simulink model "LKAS_AutoSave_DF_20220316_0937"  (R2018b)
settings: Solver=FixedStepDiscrete  StartTime=0.0  StopTime=10.0  FixedStep=0.01  RelTol=1e-3
InitFcn:
  | tmpVer = ver('MATLAB');
  | tmpVer = str2num(tmpVer.Version);
  | % -------------------------------------------------------------------
  | %  MATLAB file generated by Simulink.saveVars on 21-Nov-2019 10:06:14
  | %  MATLAB version: 7.13.0.564 (R2011b)
  | % -------------------------------------------------------------------
  | 
  | 
  | SInt16 = Simulink.AliasType;
  | SInt16.Description = 'Num';
  | if (tmpVer > 7.11)
  | 	SInt16.DataScope = 'Auto';
  | end
  | SInt16.HeaderFile = 'Rte_Type.h';
  | SInt16.BaseType = 'int16';
  | 
  | SInt32 = Simulink.AliasType;
  | SInt32.Description = 'Num';
  | if (tmpVer > 7.11)
  | 	SInt32.DataScope = 'Auto';
  | end
  | SInt32.HeaderFile = 'Rte_Type.h';
  | SInt32.BaseType = 'int32';
  | 
  | SInt8 = Simulink.AliasType;
  | SInt8.Description = 'Num';
  | if (tmpVer > 7.11)
  | 	SInt8.DataScope = 'Auto';
  | end
  | SInt8.HeaderFile = 'Rte_Type.h';
  | SInt8.BaseType = 'int8';
  | 
  | T_A_m2_1024_1_u32 = Simulink.NumericType;
  | T_A_m2_1024_1_u32.Description = 'm2 (square meters  (m2))';
  | if (tmpVer > 7.11)
  | 	T_A_m2_1024_1_u32.DataScope = 'Auto';
  | end
  | T_A_m2_1024_1_u32.HeaderFile = 'Rte_Type.h';
  | T_A_m2_1024_1_u32.DataTypeMode = 'Fixed-point: slope and bias scaling';
  | T_A_m2_1024_1_u32.SignednessBool = false;
  | T_A_m2_1024_1_u32.WordLength = 32;
  | T_A_m2_1024_1_u32.FixedExponent = -10;
  | T_A_m2_1024_1_u32.SlopeAdjustmentFactor = 1;
  | T_A_m2_1024_1_u32.Bias = 0;
  | T_A_m2_1024_1_u32.DataTypeOverride = 'Inherit';
  | T_A_m2_1024_1_u32.IsAlias = true;
  | 
  | T_A_m2_65536_1_u16 = Simulink.NumericType;
  | T_A_m2_65536_1_u16.Description = 'm2 (square meters  (m2))';
  | if (tmpVer > 7.11)
  | 	T_A_m2_65536_1_u16.DataScope = 'Auto';
  | end
  | T_A_m2_65536_1_u16.HeaderFile = 'Rte_Type.h';
  | T_A_m2_65536_1_u16.DataTypeMode = 'Fixed-point: slope and bias scaling';
  | T_A_m2_65536_1_u16.SignednessBool = false;
  | T_A_m2_65536_1_u16.WordLength = 16;
  | T_A_m2_65536_1_u16.FixedExponent = -16;
  | T_A_m2_65536_1_u16.SlopeAdjustmentFactor = 1;
  | T_A_m2_65536_1_u16.Bias = 0;
  | T_A_m2_65536_1_u16.DataTypeOverride = 'Inherit';
  | ... (+4647 lines)
StopFcn:
  | clear  T_A_m2_1024_1_u32 T_A_m2_65536_1_u16 T_A_m2_Float32 T_A_mm2_10_1_u16 T_A_mm2_4_1_s16 T_A_mm2_Float32 T_Cnt_Num_10_1_u32 T_Cnt_Num_1_1_s16 T_Cnt_Num_1_1_s32 T_Cnt_Num_1_1_s8 T_Cnt_Num_1_1_u16 T_Cnt_Num_1_1_u32 T_Cnt_Num_1_1_u8 T_E_J_1_1_s32 T_E_J_Float32 T_E_kJ_128_1_s32 T_E_kJ_Float32 T_E_kwh_10_1_u16 T_E_kwh_Float32 T_Epl_kwhpkm_100_1_u16 T_Epl_kwhpkm_Float32 T_F_N_1_1_s16 T_F_N_Float32 T_I_A_1000_1_u16 T_I_A_1048576_1_s32 T_I_A_2048_1_s16 T_I_A_32_1_s16 T_I_A_Float32 T_I_mA_1_1_s16 T_I_mA_32768_128_s16 T_I_mA_Float32 T_J_kgpm2_128_1_u16 T_J_kgpm2_Float32 T_K_NA_1000_1_s16 T_K_NA_100_1_s16 T_K_NA_100_1_u16 T_K_NA_1024_1_s16 T_K_NA_1024_1_u16 T_K_NA_128_1_s16 T_K_NA_128_1_u16 T_K_NA_128_1_u8 T_K_NA_16777216_1_u32 T_K_NA_16_1_s16 T_K_NA_16_1_u16 T_K_NA_16_1_u8 T_K_NA_1_16_u16 T_K_NA_1_1_s16 T_K_NA_1_1_u16 T_K_NA_1_1_u8 T_K_NA_32768_1_s16 T_K_NA_32768_1_u16 T_K_NA_32_1_s8 T_K_NA_4096_1_u16 T_K_NA_4194304_1_s32 T_K_NA_4194304_1_u16 T_K_NA_65536_1_s32 T_K_NA_65536_1_u16 T_K_NA_8192_1_s16 T_K_NA_8_1_s16 T_K_NA_Float32 T_M_Nm_16_1_s16 T_M_Nm_1_1_s16 T_M_Nm_32768_1_s16 T_M_Nm_32_1_s16 T_M_Nm_4_1_s16 T_M_Nm_512_1_s16 T_M_Nm_Float32 T_P_W_1_4_s16 T_P_W_1_8_s16 T_P_W_Float32 T_P_kW_128_1_s16 T_P_kW_1_8_s16 T_P_kW_8_1_s32 T_P_kW_Float32 T_Pct_pct_1024_1_s32 T_Pct_pct_1024_1_u32 T_Pct_pct_10_1_s16 T_Pct_pct_10_1_u32 T_Pct_pct_128_100_s8 T_Pct_pct_1_1_s16 T_Pct_pct_1_4_u8 T_Pct_pct_255_100_u16 T_Pct_pct_255_100_u8 T_Pct_pct_256_1_s16 T_Pct_pct_256_1_u16 T_Pct_pct_65535_100_u16 T_Pct_pct_Float32 T_R_ohm_1024_1_s16 T_R_ohm_32_1_s16 T_R_ohm_Float32 T_TK_K_16_1_s16 T_TK_K_Float32 T_T_degC_10_400_1_u16 T_T_degC_16_1_s16 T_T_degC_1_40_1_u8 T_T_degC_2_80_1_u8 T_T_degC_Float32 T_U_V_1000_1_u16 T_U_V_10_1_u8 T_U_V_200_1_u8 T_U_V_32_1_s16 T_U_V_4096_1_s16 T_U_V_512_1_s16 T_U_V_65535_8_u16 T_U_V_8192_1_u16 T_U_V_Float32 T_U_mV_1_1_s16 T_U_mV_256_20_u16 T_U_mV_Float32 T_V_l_256_1_s16 T_V_l_4096_1_s16 T_V_l_64_1_s16 T_V_l_65535_100_u16 T_V_l_Float32 T_V_ml_128_1_s16 T_V_ml_1_1_s16 T_V_ml_32768_1_s16 T_V_ml_Float32 T_V_ul_32_1_u16 T_V_ul_Float32 T_Vpl_clpkm_512_1_u16 T_Vpl_clpkm_Float32 T_a_kphps_16_1_s16 T_a_kphps_Float32 T_a_mps2_128_1_s16 T_a_mps2_Float32 T_c_MJpkg_256_1_s16 T_c_MJpkg_Float32 T_c_kJpgpK_1024_1_s16 T_c_kJpgpK_Float32 T_c_kJpkgpK_128_1_u16 T_c_kJpkgpK_Float32 T_chrg_Ah_1_1_s16 T_chrg_Ah_1_1_u16 T_chrg_Ah_1_1_u8 T_chrg_Ah_256_1_u16 T_chrg_Ah_4194304_1_s32 T_chrg_Ah_512_1_u16 T_chrg_Ah_8_1_u16 T_chrg_Ah_Float32 T_cmp_NA_100_1_s16 T_cmp_NA_128_1_s16 T_cmp_NA_16_1_s16 T_cmp_NA_32768_1_u16 T_cmp_NA_Float32 T_d2n_rpmps2_4_1_s16 T_d2n_rpmps2_Float32 T_dPct_pctps_16_1_s16 T_dPct_pctps_256_1_s16 T_dPct_pctps_Float32 T_dT_degCps_128_1_s16 T_dT_degCps_Float32 T_dV_lph_1_1_s16 T_dV_lph_Float32 T_dV_lpm_128_1_s16 T_dV_lpm_32_1_s16 T_dV_lpm_Float32 T_dV_lps_1024_1_u16 T_dV_lps_4_1_u16 T_dV_lps_Float32 T_dV_mlps_1024_1_s16 T_dV_mlps_Float32 T_d_BitField16 T_dm_gps_128_1_s16 T_dm_gps_128_1_u16 T_dm_gps_256_1_u16 T_dm_gps_Float32 T_dm_mgps_1_1_s16 T_dm_mgps_Float32 T_dn_rpmps_1_1_s16 T_dn_rpmps_2_1_s16 T_dn_rpmps_Float32 T_dp_Paps_1_1_s16 T_dp_Paps_Float32 T_dp_kPaps_1_1_s16 T_dp_kPaps_8_1_s16 T_dp_kPaps_Float32 T_dphi_degps_128_1_s16 T_dphi_degps_8_1_s16 T_dphi_degps_Float32 T_dr_ps_256_1_s16 T_dr_ps_Float32 T_drho_mgplps_1_2_s16 T_drho_mgplps_Float32 T_e_NA_1_1_u8 T_f_Hz_1_1_u16 T_f_Hz_1_1_u32 T_f_Hz_64_1_u16 T_f_Hz_8_1_s16 T_f_Hz_Float32 T_g_BitField32 T_l_km_16_1_s16 T_l_km_1_1_u16 T_l_km_1_1_u32 T_l_km_Float32 T_l_m_1024_1_s16 T_l_m_16_1_s16 T_l_m_1_1_u32 T_l_m_Float32 T_l_mm_16_1_s16 T_l_mm_1_1_u16 T_l_mm_4096_1_s16 T_l_mm_4_1_u8 T_l_mm_64_1_s16 T_l_mm_Float32 T_m_g_1_1_s16 T_m_g_2048_1_s16 T_m_g_32_1_u16 T_m_g_Float32 T_m_kg_1024_1_s16 T_m_kg_1_1_s16 T_m_kg_1_1_u32 T_m_kg_Float32 T_m_mg_128_1_s16 T_m_mg_32_1_s16 T_m_mg_Float32 T_n_rpm_1_1_s16 T_n_rpm_1_25_u8 T_n_rpm_256_50_u16 T_n_rpm_2_25_u8 T_n_rpm_4_1_u16 T_n_rpm_Float32 T_p_MPa_64_1_s16 T_p_MPa_Float32 T_p_Pa_1_1_s16 T_p_Pa_Float32 T_p_kPa_1_10_u16 T_p_kPa_1_1_s16 T_p_kPa_1_1_u8 T_p_kPa_256_1_u16 T_p_kPa_32_1_u16 T_p_kPa_64_1_s16 T_p_kPa_Float32 T_phi_deg_100_1_s16 T_phi_deg_1024_1_s16 T_phi_deg_128_1_s16 T_phi_deg_1_1_u8 T_phi_deg_256_1_s16 T_phi_deg_2_1_s8 T_phi_deg_32_1_s16 T_phi_deg_512_6_s32 T_phi_deg_Float32 T_phi_rad_2048_1_s16 T_phi_rad_Float32 T_r_NA_1024_1_s16 T_r_NA_1024_1_u16 T_r_NA_16384_1_s16 T_r_NA_16_1_s16 T_r_NA_256_1_s8 T_r_NA_256_1_u16 T_r_NA_32768_1_u16 T_r_NA_32_1_u16 T_r_NA_4096_1_s16 T_r_NA_65535_2_u16 T_r_NA_8192_1_u16 T_r_NA_Float32 T_rho_gpl_8192_1_s16 T_rho_gpl_Float32 T_rho_kgpm3_16_1_s16 T_rho_kgpm3_Float32 T_rho_mgpl_1_1_s16 T_rho_mgpl_64_1_s16 T_rho_mgpl_Float32 T_t_hour_1_1_s16 T_t_hour_Float32 T_t_m_1_1_u16 T_t_m_Float32 T_t_ms_1_1_s16 T_t_ms_1_1_u16 T_t_ms_1_1_u32 T_t_ms_4096_1_s16 T_t_ms_64_1_s16 T_t_ms_Float32 T_t_s_1000_1_s16 T_t_s_100_1_s16 T_t_s_10_1_s16 T_t_s_10_1_u16 T_t_s_1_1_s16 T_t_s_1_1_u16 T_t_s_1_1_u32 T_t_s_Float32 T_t_us_10_1_u32 T_t_us_1_1_s16 T_t_us_1_1_u32 T_t_us_1_4_u16 T_t_us_Float32 T_v_kph_1_1_u8 T_v_kph_64_1_s16 T_v_kph_64_1_u16 T_v_kph_Float32 T_v_mps_256_1_s16 T_v_mps_Float32 T_w_radps_32_1_s16 T_w_radps_Float32 T_y_BitField8 T_y_BitFieldDiagProgress T_y_BitFieldDiagStatus T_y_NA_1_1_u8 SInt16 SInt32 SInt8 T_BOOLEAN UInt16 UInt32 UInt8 s16 s32 s8 u16 u32 u8
model workspace (MAT data in the model file):
  MCOS : class17 (value not decoded)
  MCOS : class17 (value not decoded)
  MCOS : class17 (value not decoded)
  MCOS : class17 (value not decoded)
  MCOS : class17 (value not decoded)
  MCOS : class17 (value not decoded)
  MCOS : class17 (value not decoded)
  MCOS : class17 (value not decoded)
  MCOS : class17 (value not decoded)
  MCOS : class17 (value not decoded)
  MCOS : class17 (value not decoded)
  MCOS : class17 (value not decoded)
  MCOS : class17 (value not decoded)
  MCOS : class17 (value not decoded)
  MCOS : class17 (value not decoded)
  MCOS : class17 (value not decoded)
  MCOS : class17 (value not decoded)
  MCOS : class17 (value not decoded)
  MCOS : class17 (value not decoded)
  MCOS : class17 (value not decoded)
  MCOS : class17 (value not decoded)
  MCOS : class17 (value not decoded)
  MCOS : class17 (value not decoded)
  MCOS : class17 (value not decoded)
  MCOS : class17 (value not decoded)
  MCOS : class17 (value not decoded)
  MCOS : class17 (value not decoded)
  MCOS : class17 (value not decoded)
  MCOS : class17 (value not decoded)
  MCOS : class17 (value not decoded)
  MCOS : class17 (value not decoded)
  MCOS : class17 (value not decoded)
  MCOS : class17 (value not decoded)
  MCOS : class17 (value not decoded)
  MCOS : class17 (value not decoded)
  MCOS : class17 (value not decoded)
  MCOS : class17 (value not decoded)
  MCOS : class17 (value not decoded)
  MCOS : class17 (value not decoded)
  MCOS : class17 (value not decoded)
  MCOS : class17 (value not decoded)
  MCOS : class17 (value not decoded)
  MCOS : class17 (value not decoded)
  MCOS : class17 (value not decoded)
  MCOS : class17 (value not decoded)
  MCOS : class17 (value not decoded)
  MCOS : class17 (value not decoded)
  MCOS : class17 (value not decoded)
  MCOS : class17 (value not decoded)
  MCOS : class17 (value not decoded)
  MCOS : class17 (value not decoded)
  MCOS : class17 (value not decoded)
  MCOS : class17 (value not decoded)
  MCOS : class17 (value not decoded)
  MCOS : class17 (value not decoded)
  MCOS : class17 (value not decoded)
  MCOS : class17 (value not decoded)
  MCOS : class17 (value not decoded)
  MCOS : class17 (value not decoded)
  MCOS : class17 (value not decoded)
  MCOS : class17 (value not decoded)
  MCOS : class17 (value not decoded)
  MCOS : class17 (value not decoded)
  MCOS : class17 (value not decoded)
  MCOS : class17 (value not decoded)
  MCOS : class17 (value not decoded)
  MCOS : class17 (value not decoded)
  MCOS : class17 (value not decoded)
  MCOS : class17 (value not decoded)
  MCOS : class17 (value not decoded)
  MCOS : class17 (value not decoded)
  MCOS : class17 (value not decoded)
  MCOS : class17 (value not decoded)
  MCOS : class17 (value not decoded)
  MCOS : class17 (value not decoded)
  MCOS : class17 (value not decoded)
  MCOS : class17 (value not decoded)
  MCOS : class17 (value not decoded)
  MCOS : class17 (value not decoded)
  MCOS : class17 (value not decoded)
  MCOS : class17 (value not decoded)
  MCOS : class17 (value not decoded)
  MCOS : class17 (value not decoded)
  MCOS : class17 (value not decoded)
  MCOS : class17 (value not decoded)
  MCOS : class17 (value not decoded)
  MCOS : class17 (value not decoded)
  MCOS : class17 (value not decoded)
  MCOS : class17 (value not decoded)
  MCOS : class17 (value not decoded)
  MCOS : class17 (value not decoded)
  MCOS : class17 (value not decoded)
  MCOS : class17 (value not decoded)
  MCOS : class17 (value not decoded)
  MCOS : class17 (value not decoded)
  MCOS : class17 (value not decoded)
  MCOS : class17 (value not decoded)
  MCOS : class17 (value not decoded)
  MCOS : class17 (value not decoded)
  MCOS : class17 (value not decoded)
  MCOS : class17 (value not decoded)
  MCOS : class17 (value not decoded)
  MCOS : class17 (value not decoded)
  MCOS : class17 (value not decoded)
  MCOS : class17 (value not decoded)
undefined symbols (not defined in the file): LKA_CarWidth, LKA_SampleTime, LKA_StrRatio_C, LKA_Veh2CamL_C, LKA_Veh2CamW_C, LKA_WhlBaseL_C, LL_CompHdAg_C, LL_CompSWA_C, LL_CrvtPrvwT_C, LL_DesDvt_C, LL_DvtComp_C, LL_DvtPrvwT_C, LL_DvtSpdDet_vDvtSpdMin_C, LL_HandsOff_ExitTime, LL_HandsOff_TextTime, LL_HandsOff_WarnTime, LL_HdAgExT_C, LL_HdAgPrvwT_C, LL_LAccMax_C, LL_LAccRMax_C, LL_LDW_EarliestWarnLine_C, LL_LDW_LatestWarnLine_C, LL_LDWS_SUPPRESS_HEADING, LL_LFClb_TFC_FfCtlRatio_C, LL_LFClb_TFC_KdBalance_C, LL_LFClb_TFC_KdMaxSWA_C, LL_LFClb_TFC_KdV1_C, LL_LFClb_TFC_KdV2_C, LL_LFClb_TFC_KdVehSpdLwr_C, LL_LFClb_TFC_KdVehSpdUpr_C, LL_LFClb_TFC_Ki_C, LL_LFClb_TFC_KiMaxSWA_C, LL_LFClb_TFC_Kp_C, LL_LFClb_TFC_KpKlat_C, LL_LFClb_TFC_KpV1_C, LL_LFClb_TFC_KpV2_C, LL_LFClb_TFC_KpVehSpdLwr_C, LL_LFClb_TFC_KpVehSpdUpr_C, LL_LFClb_TFC_PrvwT_C, LL_LKA_EarliestWarnLine_C, LL_LKA_LatestWarnLine_C, LL_LKAExPrcs_ExitC0Dvt, LL_LKAExPrcs_ExitC0Swt, LL_LKAExPrcs_tiExitDelayTime3, LL_LKAExPrcs_tiExitTime1, LL_LKAExPrcs_tiExitTime2, LL_LKAExPrcs_tiExitTime3, LL_LKAS_OUT_OF_CONTROL_LAT_VEL, LL_LKAS_OUT_OF_CONTROL_TTLC, LL_LKASWASyn_M0, LL_LKASWASyn_M1, LL_LKASWASyn_M2, LL_LKASWASyn_M3D, LL_LKASWASyn_M3K_DT, LL_LKASWASyn_M3K_MSD, LL_LKASWASyn_SWAaddMax, LL_LKASWASyn_T2, LL_LKASWASyn_tiTrqSwaRtTime, LL_LKASWASyn_tiTrqSwaTime, LL_LKASWASyn_TrqMax ... (+46)
libraries: simulink x139, canmsglib x8, dspstat3 x3, simulink_extras x1
(part 7 of 20)

== system LKAS_AutoSave_DF_20220316_0937/LKAS/LL/LL Inputs Mapping/bsVehMovInfo ==
  bsVehMovInfoIn : Inport
  Bus Creator : BusCreator  Inputs=10
  Bus Selector2 : BusSelector  OutputSignals=ESC_LatAcc,ESC_LatAcc_Valid,ESC_YawRate,ESC_YawRate_Valid,ESC_UnYawRate,ESC_VehSpd,ESC_LonAcc,ESC_LonAcc_Valid,ESC_Brake_Press,ESC_VehSpd_Valid
  bsVehMovInfoOut : Outport
  wires:
  Bus Creator/1 -> bsVehMovInfoOut/1
  Bus Selector2/10 -> Bus Creator/10  "<ESC_VehSpd_Valid>"
  Bus Selector2/9 -> Bus Creator/9  "<ESC_Brake_Press>"
  Bus Selector2/8 -> Bus Creator/8  "<ESC_LonAcc_Valid>"
  Bus Selector2/7 -> Bus Creator/7  "<ESC_LonAcc>"
  Bus Selector2/6 -> Bus Creator/6  "<ESC_VehSpd>"
  Bus Selector2/5 -> Bus Creator/5  "<ESC_UnYawRate>"
  Bus Selector2/4 -> Bus Creator/4  "<ESC_YawRate_Valid>"
  Bus Selector2/3 -> Bus Creator/3  "<ESC_YawRate>"
  Bus Selector2/2 -> Bus Creator/2  "<ESC_LatAcc_Valid>"
  Bus Selector2/1 -> Bus Creator/1  "<ESC_LatAcc>"
  bsVehMovInfoIn/1 -> Bus Selector2/1

== system LKAS_AutoSave_DF_20220316_0937/LKAS/LL/LLOn/LDW ==
  LDW_bsLKAInfoSyn : Inport
  LDW_bsLDWClb : Inport  Port=2
  Enable : EnablePort  StatesWhenEnabling=reset  ShowOutputPort=on
      settings: AttributesFormatString=states = %<StatesWhenEnabling>
  Bus Selector : BusSelector  OutputSignals=bsHdAgInfo.phiHdAg_Lft,bsHdAgInfo.phiHdAg_Rgt
  Bus Selector1 : BusSelector  OutputSignals=bsLDWClb.LL_LDWS_SUPPRESS_HEADING,bsConstantClb.LKA_SampleTime
  Cast : DataTypeConversion  OutDataTypeStr=uint8
  Heading Angle Detection (HdAgDet) : Subsystem  Description=|
      | Block Name: Heading Angle Detection
      | Ab.: HdAgDet
      | No.: 1.3.1.0
      | Rev: 0.0.1
      | Update Date: 19-3-26
  Logical Operator : Logic  Operator=NOT  AllPortsSameDT=off  OutDataTypeStr=boolean
  Product : Product  OutDataTypeStr=uint8
  LDW_Flag : Outport  OutputWhenDisabled=reset  InitialOutput=0
      settings: AttributesFormatString=%<OutputWhenDisabled> = %<InitialOutput>
  wires:
  Logical Operator/1 -> Cast/1
  Cast/1 -> Product/2
  Bus Selector1/2 -> Heading Angle Detection (HdAgDet)/5(SampleTime)  "<LKA_SampleTime>"
  Product/1 -> LDW_Flag/1
  Heading Angle Detection (HdAgDet)/1(HdAgDet_stHdAgDetFlg) -> Logical Operator/1
  LDW_bsLKAInfoSyn/1 -> Bus Selector/1
  Enable/1 -> Heading Angle Detection (HdAgDet)/1(HdAgDet_stLDWActvFlg), Product/1
  Bus Selector/1 -> Heading Angle Detection (HdAgDet)/2(HdAgDet_phiHdAgLft)  "<phiHdAg_Lft>"
  Bus Selector/2 -> Heading Angle Detection (HdAgDet)/3(HdAgDet_phiHdAgRgt)  "<phiHdAg_Rgt>"
  LDW_bsLDWClb/1 -> Bus Selector1/1
  Bus Selector1/1 -> Heading Angle Detection (HdAgDet)/4(HdAgDet_phiHdAgThres_C)  "<LL_LDWS_SUPPRESS_HEADING>"

== system LKAS_AutoSave_DF_20220316_0937/LKAS/LL/LLOn/LKA ==
  LKA_bsInInfoSyn : Inport
  LKA_bsLKAInPInfo : Inport  Port=2
  LKA_bsLKAClb : Inport  Port=3
  Enable : EnablePort  StatesWhenEnabling=reset  ShowOutputPort=on
      settings: AttributesFormatString=states = %<StatesWhenEnabling>
  Bus Selector : BusSelector  OutputSignals=bsConstantClb.LKA_SampleTime
  Cast To Single : DataTypeConversion  OutDataTypeStr=uint8
  Driver Torque Addition (DTA) : Subsystem
  LKA Exit Processing (LKAExPrcs) : Subsystem  Description=|
      | Block Name: LKA Exit Processing 
      | Ab.: LKAExPrcs
      | No.: 1.2.2.0
      | Rev: 0.0.1
      | Update Date: 19-5-13
  "LKA Motion Planning (LKAMP) " : Subsystem  Description=|
      | Block Name: LKA Motion Planning
      | Ab.: LKAMP
      | No.: 1.2.3.0
      | Rev: 0.0.1
      | Update Date: 19-5-13
  LKA SWA Limit (LKASWALim) : Subsystem  Description=|
      | Block Name: LKA SWA Synthesis
      | Ab.: LKASWASyn
      | No.: 1.2.6.0
      | Rev: 0.0.1
      | Update Date: 19-5-13
  LKA_Mon : Subsystem
  Lane Following (LF) : Subsystem  Description=|
      | Block Name: Lane Following
      | Ab.: LF
      | No.: 02
      | Rev: 00.00.01
      | Update Date: 19-3-28
  Plan To LaneFollowing (PTLF) : Subsystem
  LKA_ExitFlg : Outport  OutputWhenDisabled=reset  InitialOutput=0
      settings: AttributesFormatString=%<OutputWhenDisabled> = %<InitialOutput>
  LKA_phiSWACmd : Outport  Port=2  OutputWhenDisabled=reset  InitialOutput=0
      settings: AttributesFormatString=%<OutputWhenDisabled> = %<InitialOutput>
  LKA_M : Outport  Port=3  OutputWhenDisabled=reset  InitialOutput=0
      settings: AttributesFormatString=%<OutputWhenDisabled> = %<InitialOutput>
  LKAMon : Outport  Port=4  OutputWhenDisabled=reset  InitialOutput=0
      settings: AttributesFormatString=%<OutputWhenDisabled> = %<InitialOutput>
  tag scope: ActFlg=global, Ff=global, LKA_ExitFlg_Mon=global, LKA_SampleTime=global, PT1=global
  wires:
  Cast To Single/1 -> [ActFlg]  "ActFlg"
  Plan To LaneFollowing (PTLF)/1(SWACmd) -> LKA SWA Limit (LKASWALim)/1(LKASWALim_phiTFCSWACmd)  "PTLFSWACmd"
  Enable/1 -> Cast To Single/1
  LKA SWA Limit (LKASWALim)/1(LKASWALim_phiSWACmd) -> LKA_phiSWACmd/1  "phiSWACmd"
  LKA Exit Processing (LKAExPrcs)/1(LKAExPrcs_stExFlg) -> LKA_ExitFlg/1, [LKA_ExitFlg_Mon]
  [Ff] -> Plan To LaneFollowing (PTLF)/5(Ff)
  [P] -> Plan To LaneFollowing (PTLF)/6(P)
  [I] -> Plan To LaneFollowing (PTLF)/7(I)
  [D] -> Plan To LaneFollowing (PTLF)/8(D)
  Driver Torque Addition (DTA)/1(DTA_phiDTASWACmd) -> [DT]  "DT"
  [DT] -> Plan To LaneFollowing (PTLF)/4(DrvTrq)
  [Plan] -> Plan To LaneFollowing (PTLF)/2(Plan)
  [PT1] -> Plan To LaneFollowing (PTLF)/3(T1)
  [PT1] -> LKA Exit Processing (LKAExPrcs)/3(LKAExPrcs_PlanT1)
  [ActFlg] -> "LKA Motion Planning (LKAMP) "/3(LKAMP_stLKAActvFlg)
  LKA_bsLKAInPInfo/1 -> [LKAInPInfo]
  [LKAInPInfo] -> "LKA Motion Planning (LKAMP) "/4(LKAMP_bsLKAInPInfo)
  [LKAInPInfo] -> LKA Exit Processing (LKAExPrcs)/1(LKAExPrcs_bsLKAInPInfo)
  [LKAInPInfo] -> Plan To LaneFollowing (PTLF)/1(InP)
  LKA_bsLKAClb/1 -> Bus Selector/1, [LKA_bsLLClb]
  [LKAInPInfo] -> LKA SWA Limit (LKASWALim)/3(LKASWALim_bsLKAInPInfo)
  [LKA_bsLLClb] -> LKA Exit Processing (LKAExPrcs)/2(LKAExPrcs_bsLKAClb)
  [LKA_bsLLClb] -> Driver Torque Addition (DTA)/2(DTA_bsLFClb)
  [LKA_bsLLClb] -> Lane Following (LF)/3(LF_bsLFClb)
  [LKA_bsLLClb] -> LKA SWA Limit (LKASWALim)/4(LKASWALim_bsLKAClb)
  LKA_bsInInfoSyn/1 -> [LKA_bsInInfoSyn]
  [LKA_bsInInfoSyn] -> "LKA Motion Planning (LKAMP) "/1(LKAMP_bsInInfoSyn)
  [LKA_bsInInfoSyn] -> Driver Torque Addition (DTA)/1(DTA_bsInInfoSyn)
  [LKA_bsInInfoSyn] -> Lane Following (LF)/1(LF_bsInInfoSyn)
  [Ff] -> LKA SWA Limit (LKASWALim)/2(LKASWALim_Ff)
  [LKAInPInfo] -> Lane Following (LF)/2(LF_bsLKAInPInfo)
  Driver Torque Addition (DTA)/2(DTA_M) -> LKA_M/1
  Lane Following (LF)/3(LF_phiIntegSWACmd) -> [I]
  Lane Following (LF)/1(LF_phiFfLFSWACmd) -> [Ff]
  Lane Following (LF)/2(LF_phiPropSWACmd) -> [P]
  Lane Following (LF)/4(LF_phiDiffSWACmd) -> [D]
  "LKA Motion Planning (LKAMP) "/1(LKAMP_phiSWACmd) -> [Plan]  "PlanSWACmd"
  "LKA Motion Planning (LKAMP) "/2(LKAMP_tiT1) -> [PT1]  "PlanT1"
  LKA_Mon/1(LKAMon) -> LKAMon/1
  [LKA_bsLLClb] -> "LKA Motion Planning (LKAMP) "/5(LKAMP_bsLLClb)
  Bus Selector/1 -> [LKA_SampleTime]  "<LKA_SampleTime>"
  [Ff] -> "LKA Motion Planning (LKAMP) "/2(LKAMP_Ff)

== system LKAS_AutoSave_DF_20220316_0937/LKAS/LL/LLOn/LKA Input Processing (LKAInP) ==
  LKAInP_bsInInfoSyn : Inport
  LKAInP_bsLLClb : Inport  Port=2
  LKAInP_ActFlg : Inport  Port=3
  Bus Creator2 : BusCreator  Inputs=10
  Curvature Calculation (Crvt) : Subsystem
  Delay : Delay  DelayLength=1
  Deviation Calculation (Dvt) : Subsystem
  Heading Angle Calculation (HdAg) : Subsystem
  Lane Width Calculation (LW) : Subsystem
  Previewed Curvature Calculation (PrCrvt) : Subsystem
  Previewed Deviation Calculation (PrDvt) : Subsystem
  Previewed Heading Angle Calculation (PrHdAg) : Subsystem
  Steering Wheel Position Calculation (SWAPosCal) : Subsystem
  TTLC Calculation (TTLCCalc) : Subsystem  Description=|
      | Block Name: TTLC Calculation
      | Ab.: TTLCCalc
      | No.: 1.1.1.1
      | Rev: 0.0.1
      | Update Date: 19-3-26
  Under The Limit (UndrLim) : Subsystem
  LKAInP_bsLKAInPInfo : Outport
  wires:
  LKAInP_bsInInfoSyn/1 -> Previewed Heading Angle Calculation (PrHdAg)/1(PrHdAg_bsInInfoSyn), TTLC Calculation (TTLCCalc)/3(TTLCCalc_bsInfo), Previewed Deviation Calculation (PrDvt)/2(PrvwDvt_bsInInfoSyn), Previewed Curvature Calculation (PrCrvt)/1(PrvwCrvt_bsInInfoSyn), Deviation Calculation (Dvt)/1(Dvt_bsInInfoSyn), Heading Angle Calculation (HdAg)/1(HdAg_bsInInfoSyn), Curvature Calculation (Crvt)/1(PrvwCrvt_bsInInfoSyn), Under The Limit (UndrLim)/1(UndrLim_bsInInfoSyn), Lane Width Calculation (LW)/1(LW_bsInInfoSyn), Steering Wheel Position Calculation (SWAPosCal)/1(SWAPosCal_bsInInfoSyn)
  [bsHdAgInfo] -> Bus Creator2/5  "bsHdAgInfo"
  LKAInP_bsLLClb/1 -> Previewed Deviation Calculation (PrDvt)/1(PrdcDvt_bsLLClb), Previewed Heading Angle Calculation (PrHdAg)/2(PrHdAg_bsLLClb), Deviation Calculation (Dvt)/2(Dvt_bsLLClb), Under The Limit (UndrLim)/2(UndrLim_bsLLClb), Steering Wheel Position Calculation (SWAPosCal)/2(SWAPosCal_bsLLClb), Previewed Curvature Calculation (PrCrvt)/2(PrvwCrvt_tiCrvtPrvwT_C), TTLC Calculation (TTLCCalc)/2(TTLCCalc_bsLLClb)
  [bsPrHdAgInfo] -> Bus Creator2/8  "bsPrHdAgInfo"
  [bsTTLCInfo] -> Bus Creator2/10  "bsTTLCInfo"
  [LaneWidth] -> Bus Creator2/1  "LaneWidth"
  [phiSWAPos] -> Bus Creator2/2  "phiSWAPos"
  [bsUndrLimInfo] -> Bus Creator2/3  "bsUndrLimInfo"
  [bsDvtInfo] -> Bus Creator2/6  "bsDvtInfo"
  [bsCrvtInfo] -> Bus Creator2/4  "bsCrvtInfo"
  [bsPrDvtInfo] -> Bus Creator2/9  "bsPrDvtInfo"
  [bsPrCrvtInfo] -> Bus Creator2/7  "bsPrCrvtInfo"
  Bus Creator2/1 -> LKAInP_bsLKAInPInfo/1
  LKAInP_ActFlg/1 -> Delay/1
  Delay/1 -> Previewed Curvature Calculation (PrCrvt)/3(PrvwCrvt_stLKAActvFlg)
  Lane Width Calculation (LW)/1(LW_LaneWidth) -> [LaneWidth]  "LaneWidth"
  Steering Wheel Position Calculation (SWAPosCal)/1(SWAPosCal) -> [phiSWAPos]  "phiSWAPos"
  Under The Limit (UndrLim)/1(UndrLim_bsUndrLimInfo) -> [bsUndrLimInfo]  "bsUndrLimInfo"
  Curvature Calculation (Crvt)/1(Crvt_bsCrvtInfo) -> [bsCrvtInfo]  "bsCrvtInfo"
  Heading Angle Calculation (HdAg)/1(HdAg_bsHdAgInfo) -> [bsHdAgInfo]  "bsHdAgInfo"
  [bsHdAgInfo] -> TTLC Calculation (TTLCCalc)/5(TTLCCalc_bsHdAgInfo)  "bsHdAgInfo"
  Deviation Calculation (Dvt)/1(Dvt_bsDvtInfo) -> [bsDvtInfo]  "bsDvtInfo"
  [bsDvtInfo] -> TTLC Calculation (TTLCCalc)/1(TTLCCalc_bsDvtInfo)  "bsDvtInfo"
  Previewed Curvature Calculation (PrCrvt)/1(PrvwCrvt_bsPrvwCrvtInfo) -> [bsPrCrvtInfo]  "bsPrCrvtInfo"
  [bsPrCrvtInfo] -> TTLC Calculation (TTLCCalc)/4(TTLCCalc_bsPrCrvtInfo)  "bsPrCrvtInfo"
  Previewed Heading Angle Calculation (PrHdAg)/1(PrHdAg_bsPrHdAgInfo) -> [bsPrHdAgInfo]  "bsPrHdAgInfo"
  Previewed Deviation Calculation (PrDvt)/1(PrvwDvt_bsPrvwDvtInfo) -> [bsPrDvtInfo]  "bsPrDvtInfo"
  TTLC Calculation (TTLCCalc)/1(TTLCCalc_bsTTLCInfo) -> [bsTTLCInfo]  "bsTTLCInfo"
  [bsTTLCInfo] -> Previewed Heading Angle Calculation (PrHdAg)/3(PrHdAg_bsTTLCInfo)  "bsTTLCInfo"

== system LKAS_AutoSave_DF_20220316_0937/LKAS/LL/LLOn/LL State Determination (LLStateDet) ==
  LLStateDet_bsInInfoSyn : Inport
  LLStateDet_bsLKAInPInfo : Inport  Port=2
  LLStateDet_bsLLClb : Inport  Port=3
  LLStateDet_stExitFlg : Inport  Port=4
  LLStateDet_SignalFault : Inport  Port=5
  Bus Creator : BusCreator  Inputs=3
  Delay : Delay  DelayLength=1
  Delay1 : Delay  DelayLength=1
  LDW_State_Machine : Stateflow chart  Description=|  TreatAsAtomicUnit=on
      | Block Name: LDW State Machine
      | Ab.: LDWSM
      | No.: 1.1.2.0
      | Rev: 0.0.1
      | Update Date: 19-3-26
      settings: RTWSystemCode=Nonreusable function
  LKA_State_Machine : Stateflow chart  Description=|  TreatAsAtomicUnit=on
      | Block Name: LKA State Machine
      | Ab.: LKASM
      | No.: 1.1.3.0
      | Rev: 0.0.1
      | Update Date: 19-3-26
      settings: RTWSystemCode=Nonreusable function
  LL State Machine Conditions (LLSMCon) : Subsystem
  LLStateDet_bsLLState : Outport
  LLStateDet_stLDWActvFlg : Outport  Port=2
  LLStateDet_stLKAActvFlg : Outport  Port=3
  Disable_Reason : Outport  Port=4
  tag scope: LDW_State_Mon=global, LKA_State_Mon=global
  wires:
  LL State Machine Conditions (LLSMCon)/2(LLSMCon_stLDWEnaCSyn) -> LDW_State_Machine/2(LDWSM_stEnaCSyn)
  LL State Machine Conditions (LLSMCon)/3(LLSMCon_stLDWDisblCSyn) -> LDW_State_Machine/3(LDWSM_stDisblCSyn)
  LL State Machine Conditions (LLSMCon)/4(LLSMCon_stLDWActvCSyn) -> LDW_State_Machine/4(LDWSM_stActvCSyn)
  LL State Machine Conditions (LLSMCon)/5(LLSMCon_stLDWDeactvCSyn) -> LDW_State_Machine/5(LDWSM_stDeactvCSyn)
  LL State Machine Conditions (LLSMCon)/1(LLSMCon_stDACMode) -> Bus Creator/2, LKA_State_Machine/1(LKASM_stLMCMode), LDW_State_Machine/1(LDWSM_stLMCMode)  "DACMode"
  LDW_State_Machine/1(LDWSM_stLDWActvFlg) -> LLStateDet_stLDWActvFlg/1
  LKA_State_Machine/1(LKASM_stLKAActvFlg) -> LLStateDet_stLKAActvFlg/1
  Delay1/1 -> LL State Machine Conditions (LLSMCon)/4(LLSMCon_bsLLState)
  Bus Creator/1 -> LLStateDet_bsLLState/1, Delay1/1  "LLState"
  LKA_State_Machine/2(LKASM_stLKAState) -> [LKA_State_Mon], Bus Creator/3  "LKA_State"
  LDW_State_Machine/2(LDWSM_stLDWState) -> [LDW_State_Mon], Bus Creator/1  "LDW_State"
  LL State Machine Conditions (LLSMCon)/6(LLSMCon_stLDWFaultCSyn) -> LDW_State_Machine/6(LDWSM_stFaultCSyn)
  LL State Machine Conditions (LLSMCon)/7(LLSMCon_stLKAEnaCSyn) -> LKA_State_Machine/2(LKASM_stEnaCSyn)
  LL State Machine Conditions (LLSMCon)/8(LLSMCon_stLKADisblCSyn) -> LKA_State_Machine/3(LKASM_stDisblCSyn)
  LL State Machine Conditions (LLSMCon)/9(LLSMCon_stLKAActvCSyn) -> LKA_State_Machine/4(LKASM_stActvCSyn)
  LL State Machine Conditions (LLSMCon)/10(LLSMCon_stLKADeactvCSyn) -> LKA_State_Machine/5(LKASM_stDeactvCSyn)
  LL State Machine Conditions (LLSMCon)/11(LLSMCon_stLKAFaultCSyn) -> LKA_State_Machine/6(LKASM_stFaultCSyn)
  LLStateDet_bsInInfoSyn/1 -> LL State Machine Conditions (LLSMCon)/1(LLSMCon_bsInInfoSyn)
  LLStateDet_bsLKAInPInfo/1 -> LL State Machine Conditions (LLSMCon)/2(LLSMCon_bsLKAInPInfo)
  LLStateDet_stExitFlg/1 -> Delay/1
  LLStateDet_bsLLClb/1 -> LL State Machine Conditions (LLSMCon)/3(LLSMCon_bsLLClb)
  Delay/1 -> LL State Machine Conditions (LLSMCon)/5(LLSMCon_stExitFlg)
  LLStateDet_SignalFault/1 -> LL State Machine Conditions (LLSMCon)/6(LLSMCon_bsSignalFault)
  LL State Machine Conditions (LLSMCon)/12(Disable_Reason) -> Disable_Reason/1

== system LKAS_AutoSave_DF_20220316_0937/LKAS/LL/LLOn/LL_Mon ==
  Disable_Reason : Inport
  LKAMon : Inport  Port=2
  Bus : BusCreator  Inputs=4
  BusInP : BusCreator  Inputs=2
  BusState : BusCreator  Inputs=2
  LLMon : Outport
  wires:
  [InPMon] -> Bus/1
  [StateMon] -> Bus/2
  LKAMon/1 -> Bus/3
  Bus/1 -> LLMon/1  "LLMon"
  [LFTTTLC_Mon] -> BusInP/1  "LFTTTLC_Mon"
  [RGTTTLC_Mon] -> BusInP/2  "RGTTTLC_Mon"
  [LDW_State_Mon] -> BusState/1  "LDW_State_Mon"
  [LKA_State_Mon] -> BusState/2  "LKA_State_Mon"
  BusInP/1 -> [InPMon]  "InPMon"
  BusState/1 -> [StateMon]  "StateMon"
  Disable_Reason/1 -> Bus/4  "Disable_Reason"

== system LKAS_AutoSave_DF_20220316_0937/LKAS/LL/LLOut/Angle2Trq ==
  LKA_Torque_Req : Inport
  Target_Angle : Inport  Port=2
  Stearing_Angle : Inport  Port=3
  Constant : Constant  Value=5  OutDataTypeStr=single
  Constant1 : Constant  Value=-5  OutDataTypeStr=single
  Constant3 : Constant  Value=5  OutDataTypeStr=single
  Constant4 : Constant  Value=-5  OutDataTypeStr=single
  Rate Limiter Dynamic : Subsystem
  Saturation Dynamic : Subsystem
  Subsystem : Subsystem
  torque : Outport  OutputWhenDisabled=reset  InitialOutput=0
  wires:
  Saturation Dynamic/1(y) -> torque/1  "Saturation_trq"
  Constant4/1 -> Saturation Dynamic/3(lo)
  Constant3/1 -> Saturation Dynamic/1(up)
  Rate Limiter Dynamic/1(Y) -> Saturation Dynamic/2(u)  "RL_trq"
  Constant1/1 -> Rate Limiter Dynamic/3(lo)
  Constant/1 -> Rate Limiter Dynamic/1(up)
  Target_Angle/1 -> Subsystem/1(Target_Angle)  "Target_Angle"
  Stearing_Angle/1 -> Subsystem/2(Stearing_Angle)  "Stearing_Angle"
  Subsystem/1(in_trq) -> Rate Limiter Dynamic/2(u)  "in_trq"
  LKA_Torque_Req/1 -> Subsystem/Enable  "LKA_Torque_Req"

== system LKAS_AutoSave_DF_20220316_0937/LKAS/LLClb/LLSMConClb/ICv to v10 ==
  In1 : Inport
  Add : Sum  Inputs=+-
  Constant : Constant  Value=2.5  OutDataTypeStr=single
  Gain : Gain  Gain=1/1.02
  Out1 : Outport
  wires:
  In1/1 -> Add/1
  Add/1 -> Gain/1
  Constant/1 -> Add/2
  Gain/1 -> Out1/1

== system LKAS_AutoSave_DF_20220316_0937/LKAS/LLClb/LLSMConClb/ICv to v11 ==
  In1 : Inport
  Add : Sum  Inputs=+-
  Constant : Constant  Value=2.5  OutDataTypeStr=single
  Gain : Gain  Gain=1/1.02
  Out1 : Outport
  wires:
  Gain/1 -> Out1/1
  Constant/1 -> Add/2
  Add/1 -> Gain/1
  In1/1 -> Add/1

== system LKAS_AutoSave_DF_20220316_0937/LKAS/LLClb/LLSMConClb/ICv to v6 ==
  In1 : Inport
  Add : Sum  Inputs=+-
  Constant : Constant  Value=2.5  OutDataTypeStr=single
  Gain : Gain  Gain=1/1.02
  Out1 : Outport
  wires:
  In1/1 -> Add/1
  Add/1 -> Gain/1
  Constant/1 -> Add/2
  Gain/1 -> Out1/1

== system LKAS_AutoSave_DF_20220316_0937/LKAS/LLClb/LLSMConClb/ICv to v7 ==
  In1 : Inport
  Add : Sum  Inputs=+-
  Constant : Constant  Value=2.5  OutDataTypeStr=single
  Gain : Gain  Gain=1/1.02
  Out1 : Outport
  wires:
  Gain/1 -> Out1/1
  Constant/1 -> Add/2
  Add/1 -> Gain/1
  In1/1 -> Add/1

== system LKAS_AutoSave_DF_20220316_0937/LKAS/LLClb/LLSMConClb/ICv to v8 ==
  In1 : Inport
  Add : Sum  Inputs=+-
  Constant : Constant  Value=2.5  OutDataTypeStr=single
  Gain : Gain  Gain=1/1.02
  Out1 : Outport
  wires:
  In1/1 -> Add/1
  Add/1 -> Gain/1
  Constant/1 -> Add/2
  Gain/1 -> Out1/1

== system LKAS_AutoSave_DF_20220316_0937/LKAS/LLClb/LLSMConClb/ICv to v9 ==
  In1 : Inport
  Add : Sum  Inputs=+-
  Constant : Constant  Value=2.5  OutDataTypeStr=single
  Gain : Gain  Gain=1/1.02
  Out1 : Outport
  wires:
  Gain/1 -> Out1/1
  Constant/1 -> Add/2
  Add/1 -> Gain/1
  In1/1 -> Add/1

== system LKAS_AutoSave_DF_20220316_0937/LKAS/LL/Human Machine Interface (HMI)/Subsystem/Sum Condition1 ==
  SampleTime : Inport
  Sum : Inport  Port=2
  state = reset : EnablePort  StatesWhenEnabling=reset
  Add1 : Sum  OutDataTypeStr=single
  Memory : Memory  InheritSampleTime=on
  Relational Operator : RelationalOperator  OutDataTypeStr=boolean  RndMeth=Nearest
  Saturation : Saturate  UpperLimit=60  LowerLimit=0
      settings: AttributesFormatString="Min = %<LowerLimit>  Max = %<UpperLimit>"
  Out : Outport  OutputWhenDisabled=reset  InitialOutput=0
      settings: AttributesFormatString=%<OutputWhenDisabled> = %<InitialOutput>
  wires:
  Memory/1 -> Add1/2
  Add1/1 -> Saturation/1
  Sum/1 -> Relational Operator/2
  Relational Operator/1 -> Out/1
  Saturation/1 -> Memory/1, Relational Operator/1
  SampleTime/1 -> Add1/1

== system LKAS_AutoSave_DF_20220316_0937/LKAS/LL/Human Machine Interface (HMI)/Subsystem/Sum Condition2 ==
  SampleTime : Inport
  Sum : Inport  Port=2
  state = reset : EnablePort  StatesWhenEnabling=reset
  Add1 : Sum  OutDataTypeStr=single
  Memory : Memory  InheritSampleTime=on
  Relational Operator : RelationalOperator  OutDataTypeStr=boolean  RndMeth=Nearest
  Saturation : Saturate  UpperLimit=60  LowerLimit=0
      settings: AttributesFormatString="Min = %<LowerLimit>  Max = %<UpperLimit>"
  Out : Outport  OutputWhenDisabled=reset  InitialOutput=0
      settings: AttributesFormatString=%<OutputWhenDisabled> = %<InitialOutput>
  wires:
  SampleTime/1 -> Add1/1
  Saturation/1 -> Relational Operator/1, Memory/1
  Relational Operator/1 -> Out/1
  Sum/1 -> Relational Operator/2
  Add1/1 -> Saturation/1
  Memory/1 -> Add1/2

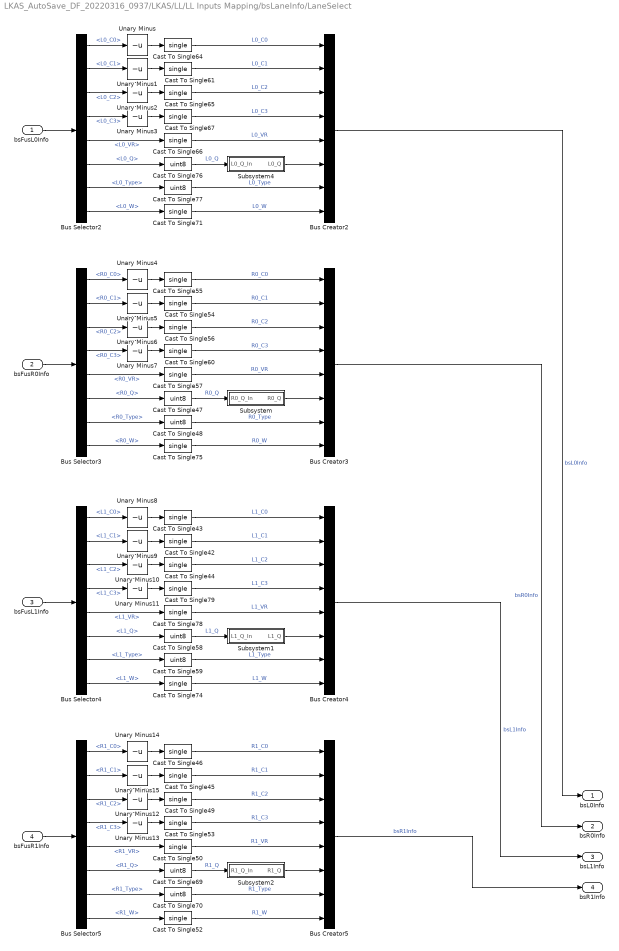
== system LKAS_AutoSave_DF_20220316_0937/LKAS/LL/LL Inputs Mapping/bsLaneInfo/LaneSelect ==
  bsFusL0Info : Inport
  bsFusR0Info : Inport  Port=2
  bsFusL1Info : Inport  Port=3
  bsFusR1Info : Inport  Port=4
  Bus Creator{2..5} (4 alike) : BusCreator  Inputs=8
  Bus Selector2 : BusSelector  OutputSignals=L0_C0,L0_C1,L0_C2,L0_C3,L0_VR,L0_Q,L0_Type,L0_W
  Bus Selector3 : BusSelector  OutputSignals=R0_C0,R0_C1,R0_C2,R0_C3,R0_VR,R0_Q,R0_Type,R0_W
  Bus Selector4 : BusSelector  OutputSignals=L1_C0,L1_C1,L1_C2,L1_C3,L1_VR,L1_Q,L1_Type,L1_W
  Bus Selector5 : BusSelector  OutputSignals=R1_C0,R1_C1,R1_C2,R1_C3,R1_VR,R1_Q,R1_Type,R1_W
  Cast To Single{42..46,49..50,52..57,60..61,64..67,71,74..75,78..79} (24 alike) : DataTypeConversion  OutDataTypeStr=single
  Cast To Single{47..48,58..59,69..70,76..77} (8 alike) : DataTypeConversion  OutDataTypeStr=uint8
  Subsystem : Subsystem
  Subsystem1 : Subsystem
  Subsystem2 : Subsystem
  Subsystem4 : Subsystem
  Unary Minus{,1..15} (16 alike) : UnaryMinus
  bsL0Info : Outport
  bsR0Info : Outport  Port=2
  bsL1Info : Outport  Port=3
  bsR1Info : Outport  Port=4
  wires:
  Bus Selector4/3 -> Unary Minus10/1  "<L1_C2>"
  Bus Selector4/8 -> Cast To Single74/1  "<L1_W>"
  Bus Selector5/3 -> Unary Minus12/1  "<R1_C2>"
  Bus Selector5/2 -> Unary Minus15/1  "<R1_C1>"
  Bus Selector5/8 -> Cast To Single52/1  "<R1_W>"
  Bus Creator5/1 -> bsR1Info/1  "bsR1Info"
  Bus Selector5/4 -> Unary Minus13/1  "<R1_C3>"
  Bus Selector3/6 -> Cast To Single47/1  "<R0_Q>"
  Subsystem/1(R0_Q) -> Bus Creator3/6
  Bus Selector2/7 -> Cast To Single77/1  "<L0_Type>"
  Bus Selector4/6 -> Cast To Single58/1  "<L1_Q>"
  Bus Selector4/4 -> Unary Minus11/1  "<L1_C3>"
  Bus Selector2/2 -> Unary Minus1/1  "<L0_C1>"
  Bus Selector3/1 -> Unary Minus4/1  "<R0_C0>"
  Bus Selector3/2 -> Unary Minus5/1  "<R0_C1>"
  Bus Selector2/8 -> Cast To Single71/1  "<L0_W>"
  Bus Selector3/4 -> Unary Minus7/1  "<R0_C3>"
  Bus Selector2/1 -> Unary Minus/1  "<L0_C0>"
  Bus Selector2/5 -> Cast To Single66/1  "<L0_VR>"
  Bus Selector5/5 -> Cast To Single50/1  "<R1_VR>"
  Bus Selector5/6 -> Cast To Single69/1  "<R1_Q>"
  Bus Selector5/7 -> Cast To Single70/1  "<R1_Type>"
  Bus Selector3/3 -> Unary Minus6/1  "<R0_C2>"
  Bus Selector3/7 -> Cast To Single48/1  "<R0_Type>"
  Bus Selector3/8 -> Cast To Single75/1  "<R0_W>"
  Bus Selector5/1 -> Unary Minus14/1  "<R1_C0>"
  Bus Selector2/3 -> Unary Minus2/1  "<L0_C2>"
  bsFusL0Info/1 -> Bus Selector2/1
  Bus Selector4/7 -> Cast To Single59/1  "<L1_Type>"
  bsFusR0Info/1 -> Bus Selector3/1
  bsFusL1Info/1 -> Bus Selector4/1
  bsFusR1Info/1 -> Bus Selector5/1
  Bus Selector2/6 -> Cast To Single76/1  "<L0_Q>"
  Bus Selector2/4 -> Unary Minus3/1  "<L0_C3>"
  Bus Selector4/1 -> Unary Minus8/1  "<L1_C0>"
  Subsystem4/1(L0_Q) -> Bus Creator2/6
  Bus Selector3/5 -> Cast To Single57/1  "<R0_VR>"
  Bus Selector4/2 -> Unary Minus9/1  "<L1_C1>"
  Bus Selector4/5 -> Cast To Single78/1  "<L1_VR>"
  Bus Creator4/1 -> bsL1Info/1  "bsL1Info"
  Bus Creator3/1 -> bsR0Info/1  "bsR0Info"
  Bus Creator2/1 -> bsL0Info/1  "bsL0Info"
  Cast To Single61/1 -> Bus Creator2/2  "L0_C1"
  Cast To Single66/1 -> Bus Creator2/5  "L0_VR"
  Cast To Single67/1 -> Bus Creator2/4  "L0_C3"
  Cast To Single65/1 -> Bus Creator2/3  "L0_C2"
  Cast To Single64/1 -> Bus Creator2/1  "L0_C0"
  Cast To Single76/1 -> Subsystem4/1(L0_Q_In)  "L0_Q"
  Cast To Single77/1 -> Bus Creator2/7  "L0_Type"
  Cast To Single56/1 -> Bus Creator3/3  "R0_C2"
  Cast To Single54/1 -> Bus Creator3/2  "R0_C1"
  Cast To Single55/1 -> Bus Creator3/1  "R0_C0"
  Cast To Single47/1 -> Subsystem/1(R0_Q_In)  "R0_Q"
  Cast To Single48/1 -> Bus Creator3/7  "R0_Type"
  Cast To Single57/1 -> Bus Creator3/5  "R0_VR"
  Cast To Single60/1 -> Bus Creator3/4  "R0_C3"
  Cast To Single75/1 -> Bus Creator3/8  "R0_W"
  Cast To Single44/1 -> Bus Creator4/3  "L1_C2"
  Cast To Single58/1 -> Subsystem1/1(L1_Q_In)  "L1_Q"
  Cast To Single59/1 -> Bus Creator4/7  "L1_Type"
  Cast To Single43/1 -> Bus Creator4/1  "L1_C0"
  Cast To Single42/1 -> Bus Creator4/2  "L1_C1"
  Cast To Single78/1 -> Bus Creator4/5  "L1_VR"
  Cast To Single79/1 -> Bus Creator4/4  "L1_C3"
  Cast To Single74/1 -> Bus Creator4/8  "L1_W"
  Cast To Single45/1 -> Bus Creator5/2  "R1_C1"
  Cast To Single46/1 -> Bus Creator5/1  "R1_C0"
  Cast To Single49/1 -> Bus Creator5/3  "R1_C2"
  Cast To Single50/1 -> Bus Creator5/5  "R1_VR"
  Cast To Single52/1 -> Bus Creator5/8  "R1_W"
  Cast To Single53/1 -> Bus Creator5/4  "R1_C3"
  Cast To Single69/1 -> Subsystem2/1(R1_Q_In)  "R1_Q"
  Cast To Single70/1 -> Bus Creator5/7  "R1_Type"
  Cast To Single71/1 -> Bus Creator2/8  "L0_W"
  Unary Minus/1 -> Cast To Single64/1
  Unary Minus1/1 -> Cast To Single61/1
  Unary Minus2/1 -> Cast To Single65/1
  Unary Minus3/1 -> Cast To Single67/1
  Unary Minus7/1 -> Cast To Single60/1
  Unary Minus6/1 -> Cast To Single56/1
  Unary Minus4/1 -> Cast To Single55/1
  Unary Minus5/1 -> Cast To Single54/1
  Unary Minus8/1 -> Cast To Single43/1
  Unary Minus9/1 -> Cast To Single42/1
  Unary Minus11/1 -> Cast To Single79/1
  Unary Minus10/1 -> Cast To Single44/1
  Unary Minus12/1 -> Cast To Single49/1
  Unary Minus13/1 -> Cast To Single53/1
  Unary Minus14/1 -> Cast To Single46/1
  Unary Minus15/1 -> Cast To Single45/1
  Subsystem1/1(L1_Q) -> Bus Creator4/6
  Subsystem2/1(R1_Q) -> Bus Creator5/6

== system LKAS_AutoSave_DF_20220316_0937/LKAS/LL/LL Inputs Mapping/bsLaneInfo/LanesReconstruct  ==
  bsLLClb : Inport
  bsL0Info : Inport  Port=2
  bsR0Info : Inport  Port=3
  bsL1Info : Inport  Port=4
  bsR1Info : Inport  Port=5
  Bus Selector5 : BusSelector  OutputSignals=L0_Q
  Bus Selector6 : BusSelector  OutputSignals=R0_Q
  LaneReconstructSM : Stateflow chart  TreatAsAtomicUnit=on
  Left 1Lane Reconstruct (Lft1LaneR) : Subsystem
  Left Lane Reconstruct (LftLaneR) : Subsystem
  Right 1Lane Reconstruct (Rgt1LaneR) : Subsystem
  Right Lane Reconstruct (RgtLaneR) : Subsystem
  RoadSide Offset : Subsystem
  Switch : Switch  Criteria=u2 > Threshold
  Switch1 : Switch  Criteria=u2 > Threshold
  bsL0InfoR : Outport
  bsR0InfoR : Outport  Port=2
  bsL1InfoR : Outport  Port=3
  bsR1InfoR : Outport  Port=4
  wires:
  bsL1Info/1 -> Left 1Lane Reconstruct (Lft1LaneR)/2(bsL1Info)
  Bus Selector6/1 -> LaneReconstructSM/2(LaneRSM_stR0Ql)  "<R0_Q>"
  Bus Selector5/1 -> LaneReconstructSM/1(LaneRSM_stL0Ql)  "<L0_Q>"
  RoadSide Offset/3(lRoadW) -> [RoadWidth], Left Lane Reconstruct (LftLaneR)/1(lRoadW), Right Lane Reconstruct (RgtLaneR)/3(lRoadW)
  Left Lane Reconstruct (LftLaneR)/1(bsL0InfoR) -> Switch1/3
  Right Lane Reconstruct (RgtLaneR)/1(bsR0InfoR) -> Switch/3
  Switch/1 -> bsR0InfoR/1
  Switch1/1 -> bsL0InfoR/1
  LaneReconstructSM/1(LaneRSM_stRoadFlg) -> [RoadFlg]
  LaneReconstructSM/2(LaneRSM_stLftFlg) -> [LftFlg]
  LaneReconstructSM/3(LaneRSM_stRgtFlg) -> [RgtFlg]
  bsR1Info/1 -> Right 1Lane Reconstruct (Rgt1LaneR)/2(bsR1Info)
  Right 1Lane Reconstruct (Rgt1LaneR)/1(bsL1InfoR) -> bsR1InfoR/1
  Left 1Lane Reconstruct (Lft1LaneR)/1(bsL1InfoR) -> bsL1InfoR/1
  [RgtFlg] -> Right 1Lane Reconstruct (Rgt1LaneR)/1(stFlag)
  [LftFlg] -> Left 1Lane Reconstruct (Lft1LaneR)/1(stFlag)
  [RgtFlg] -> Switch/2
  [LftFlg] -> Switch1/2
  bsR0Info/1 -> RoadSide Offset/2(bsR0Info)
  bsL0Info/1 -> RoadSide Offset/1(bsL0Info)
  RoadSide Offset/1(bsL0Infoout) -> Left Lane Reconstruct (LftLaneR)/3(bsL0Info), Switch1/1, Right Lane Reconstruct (RgtLaneR)/1(bsL0Info), Bus Selector5/1
  RoadSide Offset/2(bsR0Infoout) -> Switch/1, Right Lane Reconstruct (RgtLaneR)/2(bsR0Info), Left Lane Reconstruct (LftLaneR)/2(bsR0Info), Bus Selector6/1
  bsLLClb/1 -> RoadSide Offset/3(In3)

== system LKAS_AutoSave_DF_20220316_0937/LKAS/LL/LLOn/LDW/Heading Angle Detection (HdAgDet) ==
  HdAgDet_stLDWActvFlg : Inport
  HdAgDet_phiHdAgLft : Inport  Port=2
  HdAgDet_phiHdAgRgt : Inport  Port=3
  HdAgDet_phiHdAgThres_C : Inport  Port=4
  SampleTime : Inport  Port=5
  Constant : Constant  Value=0.05  OutDataTypeStr=single
  If : If  IfExpression=u1==1  ElseIfExpressions=u1==2
  If Action Subsystem : Subsystem  TreatAsAtomicUnit=on
  If Action Subsystem1 : Subsystem  TreatAsAtomicUnit=on
  If Action Subsystem2 : Subsystem  TreatAsAtomicUnit=on
  Merge : Merge  Inputs=3  InitialOutput=0
  Relational Operator : RelationalOperator  OutDataTypeStr=boolean  RndMeth=Nearest
  Sum Condition : Subsystem
  HdAgDet_stHdAgDetFlg : Outport
  wires:
  SampleTime/1 -> Sum Condition/1(In)
  If/1 -> If Action Subsystem/Action
  If Action Subsystem/1(Out1) -> Merge/1
  If Action Subsystem1/1(Out1) -> Merge/2
  If/2 -> If Action Subsystem1/Action
  If Action Subsystem2/1(Out1) -> Merge/3
  If/3 -> If Action Subsystem2/Action
  HdAgDet_phiHdAgLft/1 -> If Action Subsystem/1(In1)
  HdAgDet_phiHdAgRgt/1 -> If Action Subsystem1/1(In1)
  HdAgDet_stLDWActvFlg/1 -> If/1
  Merge/1 -> Relational Operator/1
  HdAgDet_phiHdAgThres_C/1 -> Relational Operator/2
  Relational Operator/1 -> Sum Condition/Enable
  Constant/1 -> Sum Condition/2(Sum)
  Sum Condition/1(Out) -> HdAgDet_stHdAgDetFlg/1

== system LKAS_AutoSave_DF_20220316_0937/LKAS/LL/LLOn/LKA/Driver Torque Addition (DTA) ==
  DTA_bsInInfoSyn : Inport
  DTA_bsLFClb : Inport  Port=2
  Bus Selector : BusSelector  OutputSignals=bsLKAClb.LL_LKASWAClb.LL_LKASWASyn_TrqSwaAddSwt
  Compare To Constant : simulink/Logic and Bit Operations/Compare To Constant  relop=>  const=0  OutDataTypeStr=boolean
  Driver Torque Assist : Subsystem
  Subsystem : Subsystem
  DTA_phiDTASWACmd : Outport
  DTA_M : Outport  Port=2
  wires:
  DTA_bsInInfoSyn/1 -> Subsystem/1(DTA_bsInInfoSyn), Driver Torque Assist/1(DTA_bsInInfoSyn)
  DTA_bsLFClb/1 -> Driver Torque Assist/2(DTA_bsLFClb), Bus Selector/1, Subsystem/2(DTA_bsLFClb)
  Subsystem/1(DTA_phiDTASWACmd) -> DTA_phiDTASWACmd/1
  Driver Torque Assist/1(DTA_M) -> DTA_M/1
  Bus Selector/1 -> Compare To Constant/1  "<LL_LKASWASyn_TrqSwaAddSwt>"
  Compare To Constant/1 -> Subsystem/Enable

== system LKAS_AutoSave_DF_20220316_0937/LKAS/LL/LLOn/LKA/LKA Exit Processing (LKAExPrcs) ==
  LKAExPrcs_bsLKAInPInfo : Inport
  LKAExPrcs_bsLKAClb : Inport  Port=2
  LKAExPrcs_PlanT1 : Inport  Port=3
  Cast To Single : DataTypeConversion  OutDataTypeStr=single
  Exit Time 1 : Subsystem
  Exit Time 2 : Subsystem
  Exit Time 3 : Subsystem
  Fcn : Fcn  Expr=u(3)*(u(3)==1)*3+u(2)*(u(3)==0)*2+u(1)*(u(2)==0&&u(3)==0)
  Logical Operator3 : Logic  Operator=OR  Inputs=3  AllPortsSameDT=off  OutDataTypeStr=boolean
  Mux : Mux  Inputs=3
  LKAExPrcs_stExFlg : Outport
  LKAExPrcs_stExNum : Outport  Port=2
  wires:
  Logical Operator3/1 -> LKAExPrcs_stExFlg/1
  Exit Time 1/1(Exit1) -> Mux/1, Logical Operator3/1  "Exit1"
  Exit Time 2/1(Exit2) -> Mux/2, Logical Operator3/2  "Exit2"
  Exit Time 3/1(Exit3) -> Mux/3, Logical Operator3/3  "Exit3"
  LKAExPrcs_bsLKAInPInfo/1 -> Exit Time 2/2(bsLKAInPInfo), Exit Time 3/1(bsLKAInPInfo), Exit Time 1/1(bsLKAInPInfo)
  LKAExPrcs_bsLKAClb/1 -> Exit Time 1/2(bsLKAClb), Exit Time 2/1(bsLKAClb), Exit Time 3/2(bsLKAClb)
  LKAExPrcs_PlanT1/1 -> Exit Time 2/3(T1), Exit Time 3/3(T1)
  Mux/1 -> Cast To Single/1
  Fcn/1 -> LKAExPrcs_stExNum/1  "ExNum"
  Cast To Single/1 -> Fcn/1

== system LKAS_AutoSave_DF_20220316_0937/LKAS/LL/LLOn/LKA/LKA Motion Planning (LKAMP)  ==
  LKAMP_bsInInfoSyn : Inport
  LKAMP_Ff : Inport  Port=2
  LKAMP_stLKAActvFlg : Inport  Port=3
  LKAMP_bsLKAInPInfo : Inport  Port=4
  LKAMP_bsLLClb : Inport  Port=5
  Bus Selector : BusSelector  OutputSignals=MPInP_vVehSpdIni
  Bus Selector1 : BusSelector  OutputSignals=bsVehMovInfo.ESC_VehSpd
  Bus Selector3 : BusSelector  OutputSignals=bsConstantClb.LKA_CarWidth,bsLKAClb.LL_HdAgExT_C,bsLKAClb.LL_LSpdCompT_C
  Bus Selector4 : BusSelector  OutputSignals=bsVehMovInfo.ESC_VehSpd
  Bus Selector5 : BusSelector  OutputSignals=LaneWidth
  LKA Motion Planning Calculation (LKAMPCal) : Subsystem  Description=|
      | Block Name: LKA Motion Planning Calculation
      | Ab.: LKAMPCal
      | No.: 1.2.3.2
      | Rev: 0.0.1
      | Update Date: 19-3-26
      settings: RTWSystemCode=Nonreusable function
  Motion Planning Input Processing (MPInP) : Subsystem  Description=|
      | Block Name: Motion Planning Input Processing
      | Ab.: MPInP
      | No.: 1.2.3.1
      | Rev: 0.0.1
      | Update Date: 19-3-26
  Nominal Time Calculation (NomTCalc) : Subsystem  Description=|
      | Block Name: Nominal Time Calculation
      | Ab.: NomTCalc
      | No.: 1.2.3.3
      | Rev: 0.0.1
      | Update Date: 19-3-26
  Saturation6 : Saturate  UpperLimit=2  LowerLimit=0.2
      settings: AttributesFormatString="Min = %<LowerLimit>  Max = %<UpperLimit>"
  Steering Wheel Angle Command Calculation (SWACmdCal) : Subsystem  Description=|
      | Block Name: Steering Wheel Angle Command Calculation
      | Ab.: SWACmdCal
      | No.: 1.2.3.4
      | Rev: 0.0.1
      | Update Date: 19-3-26
  Switching Condition (SwtCon) : Subsystem
  Trigger Once : Subsystem
  LKAMP_phiSWACmd : Outport
  LKAMP_tiT1 : Outport  Port=2
  wires:
  Bus Selector3/3 -> Switching Condition (SwtCon)/7(SwtCon_tiLSpdCompT_C)  "<LL_LSpdCompT_C>"
  Bus Selector3/2 -> Switching Condition (SwtCon)/6(SwtCon_tiHdAgExTime_C)  "<LL_HdAgExT_C>"
  Motion Planning Input Processing (MPInP)/1(MPInP_bsMPInPInfo) -> LKA Motion Planning Calculation (LKAMPCal)/1(LKAMPCal_bsLKAInPInfo), Steering Wheel Angle Command Calculation (SWACmdCal)/2(SWACmdCal_bsLKAInPInfo), Bus Selector/1  "LKAMP_bsMPInPInfo"
  Steering Wheel Angle Command Calculation (SWACmdCal)/2(SWACmdCal_tiT1) -> Saturation6/1
  Steering Wheel Angle Command Calculation (SWACmdCal)/1(SWACmdCal_phiSWACmd) -> LKAMP_phiSWACmd/1
  Bus Selector/1 -> Nominal Time Calculation (NomTCalc)/2(NomTCalc_vVehSpdIni)  "<MPInP_vVehSpdIni>"
  Bus Selector1/1 -> Nominal Time Calculation (NomTCalc)/1(NomTCalc_vVehSpd)  "<ESC_VehSpd>"
  Nominal Time Calculation (NomTCalc)/1(NomTCalc_tiNomT) -> Steering Wheel Angle Command Calculation (SWACmdCal)/3(SWACmdCal_tiNomT)
  Switching Condition (SwtCon)/1(SwtCon_phiHdAgMax) -> Motion Planning Input Processing (MPInP)/3(MPInP_phiHdAgMax)
  LKA Motion Planning Calculation (LKAMPCal)/1(LKAMPCal_bsLKAMPCalOut) -> Steering Wheel Angle Command Calculation (SWACmdCal)/1(SWACmdCal_bsK1K2DetOut)
  Bus Selector4/1 -> Switching Condition (SwtCon)/3(SwtCon_vVehSpd)  "<ESC_VehSpd>"
  LKAMP_stLKAActvFlg/1 -> Motion Planning Input Processing (MPInP)/2(MPInP_stLKAActvFlg), Switching Condition (SwtCon)/1(SwtCon_stLKAActvFlg)
  LKAMP_bsLLClb/1 -> LKA Motion Planning Calculation (LKAMPCal)/2(LKAMPCal_bsLKAClb), Bus Selector3/1
  LKAMP_bsLKAInPInfo/1 -> Motion Planning Input Processing (MPInP)/4(MPInP_bsLKAInPInfo), Bus Selector5/1, Switching Condition (SwtCon)/2(SwtCon_bsLKAInPInfo)
  LKAMP_bsInInfoSyn/1 -> Motion Planning Input Processing (MPInP)/5(MPInP_bsInInfoSyn), Bus Selector1/1, Bus Selector4/1
  Saturation6/1 -> LKAMP_tiT1/1
  Bus Selector5/1 -> Switching Condition (SwtCon)/4(SwtCon_lLaneWidth_C)  "<LaneWidth>"
  Bus Selector3/1 -> Switching Condition (SwtCon)/5(SwtCon_lCarWidth_C)  "<LKA_CarWidth>"
  LKAMP_Ff/1 -> Motion Planning Input Processing (MPInP)/1(MPInP_Ff)
  Trigger Once/1(Out1) -> LKA Motion Planning Calculation (LKAMPCal)/Action

== system LKAS_AutoSave_DF_20220316_0937/LKAS/LL/LLOn/LKA/LKA SWA Limit (LKASWALim) ==
  LKASWALim_phiTFCSWACmd : Inport
  LKASWALim_Ff : Inport  Port=2
  LKASWALim_bsLKAInPInfo : Inport  Port=3
  LKASWALim_bsLKAClb : Inport  Port=4
  Add : Sum  Inputs=+-+  OutDataTypeStr=single
  Add1 : Sum
  Add2 : Sum
  Bus Selector1 : BusSelector  OutputSignals=phiSWAPos,bsUndrLimInfo.UndrLim_phiSWAMax,bsUndrLimInfo.UndrLim_dphiSWARMax
  Bus Selector3 : BusSelector  OutputSignals=bsLKAClb.LL_CompSWA_C
  Gain1 : Gain  Gain=-1.4  OutDataTypeStr=single
  Gain2 : Gain  Gain=-1  OutDataTypeStr=single
  Gain3 : Gain  Gain=1.4  OutDataTypeStr=single
  "Rate Limiter Dynamic " : Subsystem
  Saturation Dynamic : simulink/Discontinuities/Saturation Dynamic  OutMin=[]  OutMax=[]  OutDataTypeStr=Inherit: Same as second input  OutDataType=fixdt(1, 16)  OutScaling=2^-10  DoSatur=off
  LKASWALim_phiSWACmd : Outport
  wires:
  Gain3/1 -> "Rate Limiter Dynamic "/1(up)
  Saturation Dynamic/1 -> "Rate Limiter Dynamic "/2(u)
  "Rate Limiter Dynamic "/1(Y) -> LKASWALim_phiSWACmd/1
  Bus Selector3/1 -> Add/2  "<LL_CompSWA_C>"
  LKASWALim_phiTFCSWACmd/1 -> Add/1
  LKASWALim_bsLKAClb/1 -> Bus Selector3/1
  Bus Selector1/2 -> Add1/2, Gain2/1  "<UndrLim_phiSWAMax>"
  Bus Selector1/3 -> Gain3/1, Gain1/1  "<UndrLim_dphiSWARMax>"
  Gain2/1 -> Add2/2
  Gain1/1 -> "Rate Limiter Dynamic "/3(lo)
  Add/1 -> Saturation Dynamic/2
  LKASWALim_bsLKAInPInfo/1 -> Bus Selector1/1
  Bus Selector1/1 -> Add/3  "<phiSWAPos>"
  LKASWALim_Ff/1 -> Add2/1, Add1/1
  Add1/1 -> Saturation Dynamic/1
  Add2/1 -> Saturation Dynamic/3

== system LKAS_AutoSave_DF_20220316_0937/LKAS/LL/LLOn/LKA/LKA_Mon ==
  BusLKA : BusCreator  Inputs=3
  CastLKA1 : DataTypeConversion  OutDataTypeStr=single
  CastLKA2 : DataTypeConversion  OutDataTypeStr=single
  CastLKA3 : DataTypeConversion  OutDataTypeStr=single
  LKAMon : Outport
  wires:
  [LKA_ExitFlg_Mon] -> CastLKA1/1
  [LKA_SampleTime_Mon] -> CastLKA2/1
  [T1_Mon] -> CastLKA3/1
  CastLKA1/1 -> BusLKA/1  "LKA_ExitFlg_Mon"
  CastLKA2/1 -> BusLKA/2  "LKA_SampleTime_Mon"
  CastLKA3/1 -> BusLKA/3  "T1_Mon"
  BusLKA/1 -> LKAMon/1  "LKAMon"
